simulink model "ParallelPIDController"  (R2018b)
settings: Solver=VariableStepAuto  StartTime=0.0  StopTime=200  RelTol=1e-3
settings Model: Creator=Alex  LastModifiedBy=Alex

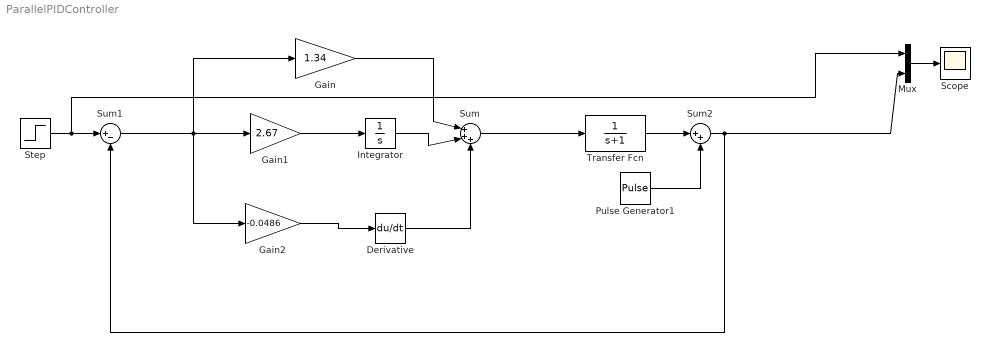
== system ParallelPIDController ==
  Derivative : Derivative
  Gain : Gain  Gain=1.34
  Gain1 : Gain  Gain=2.67
  Gain2 : Gain  Gain=-0.0486
  Integrator : Integrator
  Mux : Mux  Inputs=2
  Pulse Generator1 : DiscretePulseGenerator  PulseType=Time based  Amplitude=0.1  Period=5  PulseWidth=30
  Scope : Scope
  Step : Step  Time=0  SampleTime=0
  Sum : Sum  Inputs=|+++
  Sum1 : Sum  Inputs=|+-
  Sum2 : Sum  Inputs=|++
  Transfer Fcn : TransferFcn  Denominator=[1 1]
  wires:
  Gain1/1 -> Integrator/1
  Gain2/1 -> Derivative/1
  Gain/1 -> Sum/1
  Integrator/1 -> Sum/2
  Derivative/1 -> Sum/3
  Sum/1 -> Transfer Fcn/1
  Sum1/1 -> Gain/1, Gain1/1, Gain2/1
  Mux/1 -> Scope/1
  Transfer Fcn/1 -> Sum2/1
  Pulse Generator1/1 -> Sum2/2
  Step/1 -> Mux/1, Sum1/1
  Sum2/1 -> Sum1/2, Mux/2
